simulink model "SOH_OL_Harness"  (R2015b)
settings: Solver=FixedStepAuto  StartTime=0.0  StopTime=sim_time  FixedStep=sample_time  RelTol=1e-3
libraries: simulink x1
settings Model: Creator=favv5g  LastModifiedBy=favv5g

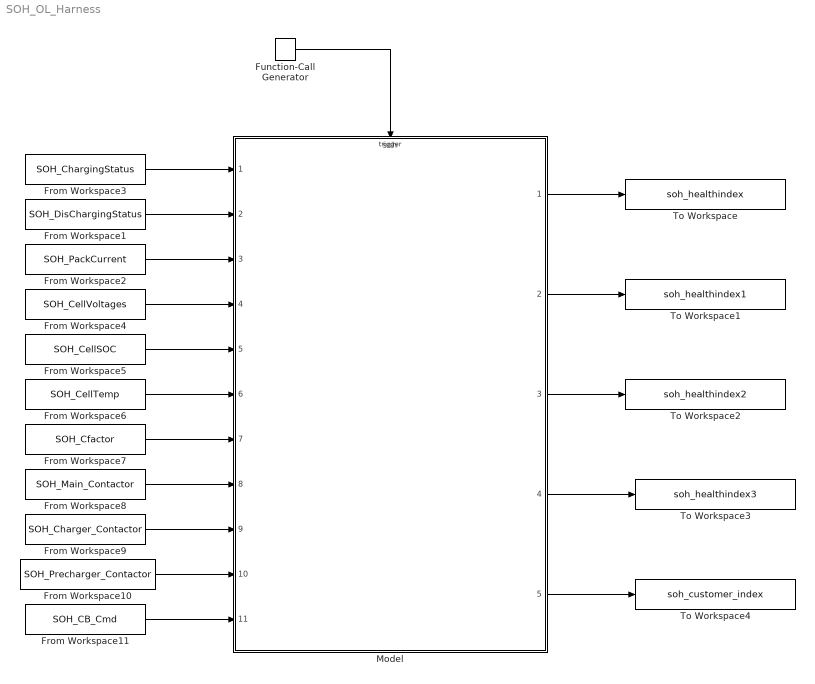
== system SOH_OL_Harness ==
  From Workspace1 : FromWorkspace  VariableName=SOH_DisChargingStatus
  From Workspace10 : FromWorkspace  VariableName=SOH_Precharger_Contactor
  From Workspace11 : FromWorkspace  VariableName=SOH_CB_Cmd
  From Workspace2 : FromWorkspace  VariableName=SOH_PackCurrent
  From Workspace3 : FromWorkspace  VariableName=SOH_ChargingStatus
  From Workspace4 : FromWorkspace  VariableName=SOH_CellVoltages
  From Workspace5 : FromWorkspace  VariableName=SOH_CellSOC
  From Workspace6 : FromWorkspace  VariableName=SOH_CellTemp
  From Workspace7 : FromWorkspace  VariableName=SOH_Cfactor
  From Workspace8 : FromWorkspace  VariableName=SOH_Main_Contactor
  From Workspace9 : FromWorkspace  VariableName=SOH_Charger_Contactor
  Function-Call Generator : simulink/Ports & Subsystems/Function-Call Generator  sample_time=0.01  numberOfIterations=1
  Model : ModelReference  ModelNameDialog=soh.slx  SimulationMode=Normal  ModelReferenceVersion=1.260  CopyOfModelName=soh.slx  TriggerPortName=Trigger  TriggerPortTriggerType=function-call  TriggerPortStatesWhenEnabling=held
  To Workspace : ToWorkspace  VariableName=soh_healthindex  SaveFormat=Timeseries  SampleTime=-1
  To Workspace1 : ToWorkspace  VariableName=soh_healthindex1  SaveFormat=Timeseries  SampleTime=-1
  To Workspace2 : ToWorkspace  VariableName=soh_healthindex2  SaveFormat=Timeseries  SampleTime=-1
  To Workspace3 : ToWorkspace  VariableName=soh_healthindex3  SaveFormat=Timeseries  SampleTime=-1
  To Workspace4 : ToWorkspace  VariableName=soh_customer_index  SaveFormat=Timeseries  SampleTime=-1
  wires:
  From Workspace3/1 -> Model/1
  From Workspace1/1 -> Model/2
  From Workspace2/1 -> Model/3
  From Workspace4/1 -> Model/4
  From Workspace5/1 -> Model/5
  From Workspace6/1 -> Model/6
  Model/1 -> To Workspace/1
  Function-Call Generator/1 -> Model/Trigger
  From Workspace7/1 -> Model/7
  Model/2 -> To Workspace1/1
  Model/3 -> To Workspace2/1
  Model/4 -> To Workspace3/1
  From Workspace8/1 -> Model/8
  From Workspace9/1 -> Model/9
  From Workspace10/1 -> Model/10
  From Workspace11/1 -> Model/11
  Model/5 -> To Workspace4/1
